simulink model "T_101"  (R2023a)
settings: Solver=VariableStepAuto  StartTime=0.0  StopTime=inf  RelTol=1e-3
settings Model: Creator=JesseJabezArendse  LastModifiedBy=JesseJabezArendse

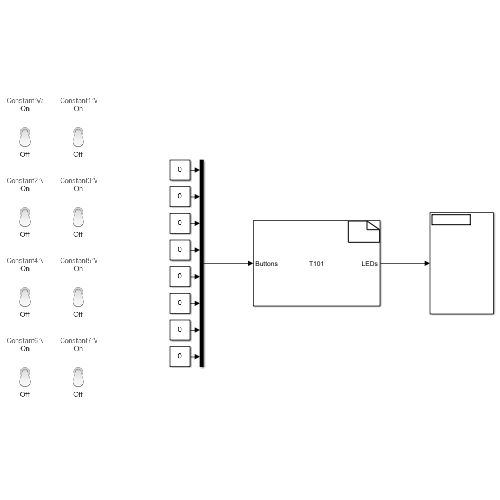
[thumbnail: Simulink's stored preview of the top-level diagram]
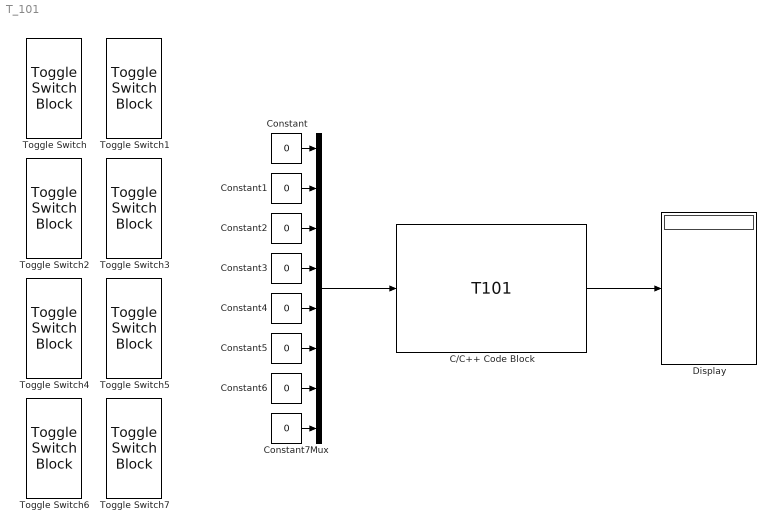
== system T_101 ==
  C/C++ Code Block : S-Function  FunctionName=T101  SFunctionModules=T101_wrapper.cpp  SFunctionDeploymentMode=off  EnableBusSupport=off  mask(S-Function Builder){}
      mask help: Simulink:masks:SFunctionBuilder_MD
      mask init:
      | val = [[.9  0.75 0.75 1 1 .9 .9 1]',[1 1 0.75 0.75 .9 .9 1 .9]'];try , sys = get_param(gcb,'SfunBuilderFcnName');if isempty(sys), sys = get_param(gcb,'FunctionName'); end,catch, sys = get_param(gcb,'FunctionName'); end
      settings: CopyFcn=set_param(gcbh,'LinkStatus','none')  OpenFcn=sfunctionwizard(gcbh)
      mask Display:
      | plot(val(:,1),val(:,2))
      | disp(sys)
      | port_label('input',1,'Buttons')
      | port_label('output',1,'LEDs')
  Constant{,1..7} (8 alike) : Constant  Value=0
  Display : Display
  Mux : Mux  Inputs=8
  Toggle Switch{,1..7} (8 alike) : ToggleSwitchBlock
      settings: Values={{'Off', 'On'}, [0 1]}
  wires:
  Constant6/1 -> Mux/7
  Constant7/1 -> Mux/8
  Constant5/1 -> Mux/6
  Constant4/1 -> Mux/5
  Constant3/1 -> Mux/4
  Constant/1 -> Mux/1
  Constant1/1 -> Mux/2
  Constant2/1 -> Mux/3
  C/C++ Code Block/1 -> Display/1
  Mux/1 -> C/C++ Code Block/1
